simulink library "uav_utilities"  (Simulink 7.1)
values from neighbouring files (symbols this model uses):
  I = find(Ev == Ev(1))    [res_power_junction_m.m]
undefined symbols (not defined in the file or in its folder): euler_0, g, inner_sysd, K_inner, K_outer, Kx_inner, KX_outer, Ky_inner, KY_outer, L, m, omega_0, outer_sysd, pow_gps_pos_sim, pow_gps_vel_sim, pow_imu_pos_sim, pow_imu_rate_sim, pow_sodar_sim, t_comp_inner, t_comp_outer, t_gps, t_imu, t_inner, t_outer, t_sodar, tau, thrust_max, torque_max, Vb_0, XYZ_0
libraries: simulink x33, aero_sim_lib x9, aerolibprivatev1p5 x1
(part 2 of 3)

== system uav_utilities/STARMAC/starmac_dynamics/starmac_motor_dynamics ==
  desired_motor_thrust : Inport  OutDataType=sfix(16)  OutScaling=2^0
  Band-Limited White Noise : simulink/Sources/Band-Limited White Noise  SystemSampleTime=-1  Cov=Ts*motor_variance*ones(4,1)  Ts=Ts  seed=22341+[0 1 2 3]'
  Constant : Constant  Value=motor_lag_enable  OutDataType=sfix(16)  OutScaling=2^0
  Saturation : Saturate  UpperLimit=thrust_max*ones(4,1)  LowerLimit=thrust_min*ones(4,1)
  State-Space : StateSpace  A=-(1/tau_motor)*eye(4)  B=(1/tau_motor)*eye(4)  C=eye(4)  D=zeros(4,4)  X0=T_nom*ones(4,1)
  Sum : Sum  Inputs=|++  OutDataType=sfix(16)  OutScaling=2^0
  Switch : Switch  Criteria=u2 > Threshold  OutDataType=sfix(16)  OutScaling=2^0
  motor_thrust : Outport  OutDataType=sfix(16)  OutScaling=2^0
  wires:
  Constant/1 -> Switch/2
  Switch/1 -> Saturation/1
  State-Space/1 -> Switch/1
  Band-Limited White Noise/1 -> Sum/2
  Saturation/1 -> Sum/1
  Sum/1 -> motor_thrust/1
  desired_motor_thrust/1 -> Switch/3, State-Space/1

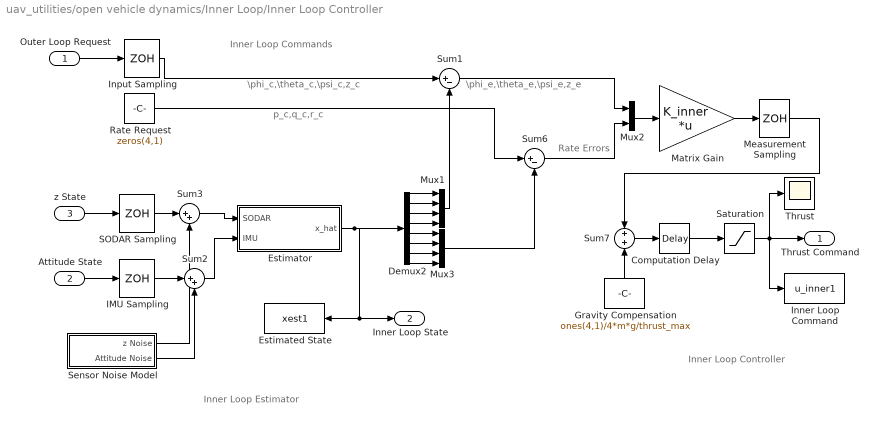
== system uav_utilities/open vehicle dynamics/Inner Loop/Inner Loop Controller ==
  note: \phi_e,\theta_e,\psi_e,z_e
  note: Rate Errors
  note: \phi_c,\theta_c,\psi_c,z_c
  note: Inner Loop Controller
  note: p_c,q_c,r_c
  note: Inner Loop Estimator
  note: Inner Loop Commands
  Outer Loop Request : Inport  OutDataType=sfix(16)  OutScaling=2^0
  Attitude State : Inport  Port=2  OutDataType=sfix(16)  OutScaling=2^0
  z State : Inport  Port=3  OutDataType=sfix(16)  OutScaling=2^0
  Computation Delay : TransportDelay  DelayTime=t_comp_inner  PadeOrder=10
  Demux2 : Demux  Outputs=8
  Estimated State : ToWorkspace  VariableName=xest1  SampleTime=-1  SaveFormat=Array
  Estimator : Subsystem
  Gravity Compensation : Constant  Orientation=up  Value=ones(4,1)/4*m*g/thrust_max  OutDataType=sfix(16)  OutScaling=2^0
  IMU Sampling : ZeroOrderHold  SampleTime=t_imu
  Inner Loop Command : ToWorkspace  VariableName=u_inner1  SampleTime=-1  SaveFormat=Array
  Input Sampling : ZeroOrderHold  SampleTime=t_inner
  Matrix Gain : Gain  Gain=K_inner  Multiplication=Matrix(K*u)  ParameterDataType=sfix(16)  ParameterScaling=2^0  OutDataType=sfix(16)  OutScaling=2^0  SaturateOnIntegerOverflow=on  OutDataTypeStr=Inherit: Same as input  ParamDataTypeStr=Inherit: Same as input
  Measurement Sampling : ZeroOrderHold  SampleTime=t_inner
  Mux1 : Mux
  Mux2 : Mux  Inputs=2
  Mux3 : Mux
  Rate Request : Constant  Value=zeros(4,1)  OutDataType=sfix(16)  OutScaling=2^0
  SODAR Sampling : ZeroOrderHold  SampleTime=t_sodar
  Saturation : Saturate  UpperLimit=1  LowerLimit=0
  "Sensor Noise Model  " : Subsystem
  Sum1 : Sum  Inputs=|+-  OutDataType=sfix(16)  OutScaling=2^0  SaturateOnIntegerOverflow=on
  Sum2 : Sum  Inputs=|++  OutDataType=sfix(16)  OutScaling=2^0  SaturateOnIntegerOverflow=on
  Sum3 : Sum  Inputs=|++  OutDataType=sfix(16)  OutScaling=2^0  SaturateOnIntegerOverflow=on
  Sum6 : Sum  Inputs=|+-  OutDataType=sfix(16)  OutScaling=2^0  SaturateOnIntegerOverflow=on
  Sum7 : Sum  OutDataType=sfix(16)  OutScaling=2^0  SaturateOnIntegerOverflow=on
  Thrust : Scope
      settings: SaveName=ScopeData7
  Thrust Command : Outport  OutDataType=sfix(16)  OutScaling=2^0
  Inner Loop State : Outport  Port=2  OutDataType=sfix(16)  OutScaling=2^0
  wires:
  Attitude State/1 -> IMU Sampling/1
  Sum1/1 -> Mux2/1
  Mux2/1 -> Matrix Gain/1
  Matrix Gain/1 -> Measurement Sampling/1
  z State/1 -> SODAR Sampling/1
  Mux1/1 -> Sum1/2
  Gravity Compensation/1 -> Sum7/2
  Sum7/1 -> Computation Delay/1
  Outer Loop Request/1 -> Input Sampling/1
  Input Sampling/1 -> Sum1/1
  Measurement Sampling/1 -> Sum7/1
  Demux2/3 -> Mux1/3
  Demux2/2 -> Mux1/2
  Demux2/1 -> Mux1/1
  Demux2/4 -> Mux1/4
  Sum6/1 -> Mux2/2
  Rate Request/1 -> Sum6/1
  Mux3/1 -> Sum6/2
  Demux2/5 -> Mux3/1
  Demux2/6 -> Mux3/2
  Demux2/7 -> Mux3/3
  Demux2/8 -> Mux3/4
  Estimator/1(x_hat) -> Demux2/1, Estimated State/1, Inner Loop State/1
  Sum2/1 -> Estimator/2(IMU)
  SODAR Sampling/1 -> Sum3/1
  Sum3/1 -> Estimator/1(SODAR)
  IMU Sampling/1 -> Sum2/1
  Saturation/1 -> Thrust Command/1, Inner Loop Command/1, Thrust/1
  Computation Delay/1 -> Saturation/1
  "Sensor Noise Model  "/1(z Noise) -> Sum3/2
  "Sensor Noise Model  "/2(Attitude Noise) -> Sum2/2

== system uav_utilities/open vehicle dynamics/Inner Loop/Non-Linear Dynamics ==
  Thrust Command 1-4 : Inport  OutDataType=sfix(16)  OutScaling=2^0
  6DOF (Euler Angles)_CMU : aero_sim_lib/6DOF (Euler Angles)_CMU  SystemSampleTime=-1  XYZe_0=XYZ_0  Vb_0=Vb_0  euler_0=euler_0  omega_0=omega_0  M=m  I=I
  Gravity : Constant  Value=[0;0;-m*g]  OutDataType=sfix(16)  OutScaling=2^0
  Motor Model : Subsystem
  Rotational Torques : Subsystem
  Sum : Sum  Inputs=|++  OutDataType=sfix(16)  OutScaling=2^0  SaturateOnIntegerOverflow=on
  Terminator : Terminator
  Terminator1 : Terminator
  Terminator2 : Terminator
  "Body vel " : Outport  OutDataType=sfix(16)  OutScaling=2^0
  Position : Outport  Port=2  OutDataType=sfix(16)  OutScaling=2^0
  Velocity : Outport  Port=3  OutDataType=sfix(16)  OutScaling=2^0
  Angular Rates : Outport  Port=4  OutDataType=sfix(16)  OutScaling=2^0
  Euler Angles : Outport  Port=5  OutDataType=sfix(16)  OutScaling=2^0
  wires:
  Thrust Command 1-4/1 -> Motor Model/1(Thrust Command 1-4), Rotational Torques/1(Thrust Command 1-4)
  Rotational Torques/1(Moments) -> 6DOF (Euler Angles)_CMU/2
  6DOF (Euler Angles)_CMU/1 -> Velocity/1
  6DOF (Euler Angles)_CMU/2 -> Position/1
  6DOF (Euler Angles)_CMU/5 -> "Body vel "/1
  6DOF (Euler Angles)_CMU/3 -> Motor Model/2(Euler (rad)), Euler Angles/1
  6DOF (Euler Angles)_CMU/6 -> Angular Rates/1
  6DOF (Euler Angles)_CMU/4 -> Terminator1/1
  6DOF (Euler Angles)_CMU/7 -> Terminator/1
  Motor Model/1("Force_b ") -> Sum/1
  Gravity/1 -> Sum/2
  Sum/1 -> 6DOF (Euler Angles)_CMU/1
  6DOF (Euler Angles)_CMU/8 -> Terminator2/1

== system uav_utilities/open vehicle dynamics/Inner Loop/Saturation ==
  note: No longer saturating
      | the z cordinate??!!!XXX
      | was set from 0 to 3
      | Nicholas Kottenstette
  Actual : Inport  OutDataType=sfix(16)  OutScaling=2^0
  Demux : Demux  Outputs=3
  Mux : Mux  Inputs=3
  Sensed : Outport  OutDataType=sfix(16)  OutScaling=2^0
  wires:
  Actual/1 -> Demux/1
  Mux/1 -> Sensed/1
  Demux/2 -> Mux/2
  Demux/1 -> Mux/1
  Demux/3 -> Mux/3

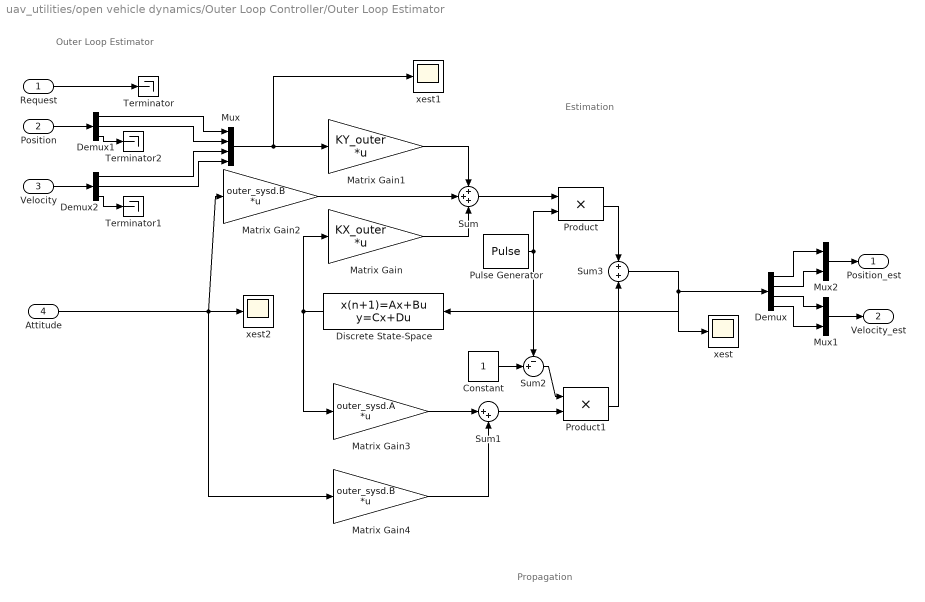
== system uav_utilities/open vehicle dynamics/Outer Loop Controller/Outer Loop Estimator ==
  note: Outer Loop Estimator
  note: Estimation
  note: Propagation
  Request : Inport  OutDataType=sfix(16)  OutScaling=2^0
  Position : Inport  Port=2  OutDataType=sfix(16)  OutScaling=2^0
  Velocity : Inport  Port=3  OutDataType=sfix(16)  OutScaling=2^0
  Attitude : Inport  Port=4  OutDataType=sfix(16)  OutScaling=2^0
  Constant : Constant  OutDataType=sfix(16)  OutScaling=2^0
  Demux : Demux
  Demux1 : Demux  Outputs=3
  Demux2 : Demux  Outputs=3
  Discrete State-Space : DiscreteStateSpace  Orientation=left  A=zeros(4)  B=eye(4)  C=eye(4)  D=zeros(4)  X0=zeros(4,1)  SampleTime=t_outer
  Matrix Gain : Gain  Gain=KX_outer  Multiplication=Matrix(K*u)  ParameterDataType=sfix(16)  ParameterScaling=2^0  OutDataType=sfix(16)  OutScaling=2^0  SaturateOnIntegerOverflow=on  OutDataTypeStr=Inherit: Same as input  ParamDataTypeStr=Inherit: Same as input
  Matrix Gain1 : Gain  Gain=KY_outer  Multiplication=Matrix(K*u)  ParameterDataType=sfix(16)  ParameterScaling=2^0  OutDataType=sfix(16)  OutScaling=2^0  SaturateOnIntegerOverflow=on  OutDataTypeStr=Inherit: Same as input  ParamDataTypeStr=Inherit: Same as input
  Matrix Gain2 : Gain  Gain=outer_sysd.B  Multiplication=Matrix(K*u)  ParameterDataType=sfix(16)  ParameterScaling=2^0  OutDataType=sfix(16)  OutScaling=2^0  SaturateOnIntegerOverflow=on  OutDataTypeStr=Inherit: Same as input  ParamDataTypeStr=Inherit: Same as input
  Matrix Gain3 : Gain  Gain=outer_sysd.A  Multiplication=Matrix(K*u)  ParameterDataType=sfix(16)  ParameterScaling=2^0  OutDataType=sfix(16)  OutScaling=2^0  SaturateOnIntegerOverflow=on  OutDataTypeStr=Inherit: Same as input  ParamDataTypeStr=Inherit: Same as input
  Matrix Gain4 : Gain  Gain=outer_sysd.B  Multiplication=Matrix(K*u)  ParameterDataType=sfix(16)  ParameterScaling=2^0  OutDataType=sfix(16)  OutScaling=2^0  SaturateOnIntegerOverflow=on  OutDataTypeStr=Inherit: Same as input  ParamDataTypeStr=Inherit: Same as input
  Mux : Mux
  Mux1 : Mux  Inputs=2
  Mux2 : Mux  Inputs=2
  Product : Product  OutDataType=sfix(16)  OutScaling=2^0  SaturateOnIntegerOverflow=on  OutDataTypeStr=Inherit: Same as first input
  Product1 : Product  OutDataType=sfix(16)  OutScaling=2^0  SaturateOnIntegerOverflow=on  OutDataTypeStr=Inherit: Same as first input
  Pulse Generator : DiscretePulseGenerator  PulseType=Time based  Period=t_gps  PulseWidth=100*t_outer/t_gps
  Sum : Sum  Inputs=+++  OutDataType=sfix(16)  OutScaling=2^0  SaturateOnIntegerOverflow=on
  Sum1 : Sum  Inputs=|++  OutDataType=sfix(16)  OutScaling=2^0  SaturateOnIntegerOverflow=on
  Sum2 : Sum  Inputs=-+|  OutDataType=sfix(16)  OutScaling=2^0  SaturateOnIntegerOverflow=on
  Sum3 : Sum  OutDataType=sfix(16)  OutScaling=2^0  SaturateOnIntegerOverflow=on
  Terminator : Terminator
  Terminator1 : Terminator
  Terminator2 : Terminator
  xest : Scope
      settings: Decimation=10
  xest1 : Scope
      settings: SaveName=ScopeData9  Decimation=10
  xest2 : Scope
      settings: SaveName=ScopeData10
  Position_est : Outport  OutDataType=sfix(16)  OutScaling=2^0
  Velocity_est : Outport  Port=2  OutDataType=sfix(16)  OutScaling=2^0
  wires:
  Request/1 -> Terminator/1
  Matrix Gain1/1 -> Sum/1
  Sum/1 -> Product/1
  Matrix Gain/1 -> Sum/3
  Matrix Gain2/1 -> Sum/2
  Discrete State-Space/1 -> Matrix Gain/1, Matrix Gain3/1
  Mux/1 -> Matrix Gain1/1, xest1/1
  Mux1/1 -> Velocity_est/1
  Mux2/1 -> Position_est/1
  Demux/1 -> Mux2/1
  Demux/2 -> Mux2/2
  Demux/3 -> Mux1/1
  Demux/4 -> Mux1/2
  Position/1 -> Demux1/1
  Velocity/1 -> Demux2/1
  Demux2/3 -> Terminator1/1
  Demux1/3 -> Terminator2/1
  Demux2/1 -> Mux/3
  Demux2/2 -> Mux/4
  Demux1/2 -> Mux/2
  Demux1/1 -> Mux/1
  Attitude/1 -> Matrix Gain2/1, xest2/1, Matrix Gain4/1
  Matrix Gain4/1 -> Sum1/2
  Matrix Gain3/1 -> Sum1/1
  Pulse Generator/1 -> Product/2, Sum2/1
  Product/1 -> Sum3/1
  Constant/1 -> Sum2/2
  Sum2/1 -> Product1/1
  Sum1/1 -> Product1/2
  Product1/1 -> Sum3/2
  Sum3/1 -> Demux/1, Discrete State-Space/1, xest/1

== system uav_utilities/open vehicle dynamics/Outer Loop Controller/Sensor Noise Model  ==
  Mux1 : Mux  Inputs=3
  Mux3 : Mux  Inputs=3
  Vx White Noise : simulink/Sources/Band-Limited White Noise  SystemSampleTime=-1  Cov=[pow_gps_vel_sim]  Ts=t_gps  seed=[2]
  Vy White Noise : simulink/Sources/Band-Limited White Noise  SystemSampleTime=-1  Cov=[pow_gps_vel_sim]  Ts=t_gps  seed=[500]
  Vz White Noise : simulink/Sources/Band-Limited White Noise  SystemSampleTime=-1  Cov=[pow_gps_vel_sim]  Ts=t_gps  seed=[1000]
  x White Noise : simulink/Sources/Band-Limited White Noise  SystemSampleTime=-1  Cov=[pow_gps_pos_sim]  Ts=t_gps  seed=[13341]
  y White Noise : simulink/Sources/Band-Limited White Noise  SystemSampleTime=-1  Cov=[pow_gps_pos_sim]  Ts=t_gps  seed=[23121]
  z White Noise1 : simulink/Sources/Band-Limited White Noise  SystemSampleTime=-1  Cov=[pow_gps_pos_sim]  Ts=t_gps  seed=[53341]
  Position Noise : Outport  OutDataType=sfix(16)  OutScaling=2^0
  Velocity Noise : Outport  Port=2  OutDataType=sfix(16)  OutScaling=2^0
  wires:
  Mux3/1 -> Position Noise/1
  z White Noise1/1 -> Mux3/3
  y White Noise/1 -> Mux3/2
  x White Noise/1 -> Mux3/1
  Mux1/1 -> Velocity Noise/1
  Vz White Noise/1 -> Mux1/3
  Vy White Noise/1 -> Mux1/2
  Vx White Noise/1 -> Mux1/1

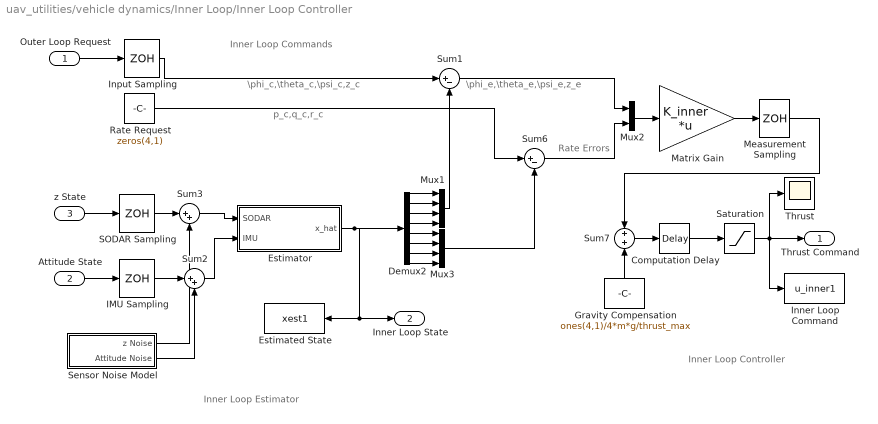
== system uav_utilities/vehicle dynamics/Inner Loop/Inner Loop Controller ==
  note: Inner Loop Commands
  note: Inner Loop Estimator
  note: p_c,q_c,r_c
  note: Inner Loop Controller
  note: \phi_c,\theta_c,\psi_c,z_c
  note: Rate Errors
  note: \phi_e,\theta_e,\psi_e,z_e
  Outer Loop Request : Inport
  Attitude State : Inport  Port=2
  z State : Inport  Port=3
  Computation Delay : TransportDelay  DelayTime=t_comp_inner  PadeOrder=10
  Demux2 : Demux  Outputs=8
  Estimated State : ToWorkspace  VariableName=xest1  SampleTime=-1  SaveFormat=Array
  Estimator : Subsystem
  Gravity Compensation : Constant  Orientation=up  Value=ones(4,1)/4*m*g/thrust_max
  IMU Sampling : ZeroOrderHold  SampleTime=t_imu
  Inner Loop Command : ToWorkspace  VariableName=u_inner1  SampleTime=-1  SaveFormat=Array
  Input Sampling : ZeroOrderHold  SampleTime=t_inner
  Matrix Gain : Gain  Gain=K_inner  Multiplication=Matrix(K*u)  SaturateOnIntegerOverflow=on  OutDataTypeStr=Inherit: Same as input  ParamDataTypeStr=Inherit: Same as input
  Measurement Sampling : ZeroOrderHold  SampleTime=t_inner
  Mux1 : Mux
  Mux2 : Mux  Inputs=2
  Mux3 : Mux
  Rate Request : Constant  Value=zeros(4,1)
  SODAR Sampling : ZeroOrderHold  SampleTime=t_sodar
  Saturation : Saturate  UpperLimit=1  LowerLimit=0
  "Sensor Noise Model  " : Subsystem
  Sum1 : Sum  Inputs=|+-  SaturateOnIntegerOverflow=on
  Sum2 : Sum  Inputs=|++  SaturateOnIntegerOverflow=on
  Sum3 : Sum  Inputs=|++  SaturateOnIntegerOverflow=on
  Sum6 : Sum  Inputs=|+-  SaturateOnIntegerOverflow=on
  Sum7 : Sum  SaturateOnIntegerOverflow=on
  Thrust : Scope
      settings: SaveName=ScopeData7
  Thrust Command : Outport
  Inner Loop State : Outport  Port=2
  wires:
  "Sensor Noise Model  "/2(Attitude Noise) -> Sum2/2
  "Sensor Noise Model  "/1(z Noise) -> Sum3/2
  Computation Delay/1 -> Saturation/1
  Saturation/1 -> Thrust/1, Inner Loop Command/1, Thrust Command/1
  IMU Sampling/1 -> Sum2/1
  Sum3/1 -> Estimator/1(SODAR)
  SODAR Sampling/1 -> Sum3/1
  Sum2/1 -> Estimator/2(IMU)
  Estimator/1(x_hat) -> Inner Loop State/1, Estimated State/1, Demux2/1
  Demux2/8 -> Mux3/4
  Demux2/7 -> Mux3/3
  Demux2/6 -> Mux3/2
  Demux2/5 -> Mux3/1
  Mux3/1 -> Sum6/2
  Rate Request/1 -> Sum6/1
  Sum6/1 -> Mux2/2
  Demux2/4 -> Mux1/4
  Demux2/1 -> Mux1/1
  Demux2/2 -> Mux1/2
  Demux2/3 -> Mux1/3
  Measurement Sampling/1 -> Sum7/1
  Input Sampling/1 -> Sum1/1
  Outer Loop Request/1 -> Input Sampling/1
  Sum7/1 -> Computation Delay/1
  Gravity Compensation/1 -> Sum7/2
  Mux1/1 -> Sum1/2
  z State/1 -> SODAR Sampling/1
  Matrix Gain/1 -> Measurement Sampling/1
  Mux2/1 -> Matrix Gain/1
  Sum1/1 -> Mux2/1
  Attitude State/1 -> IMU Sampling/1

== system uav_utilities/vehicle dynamics/Inner Loop/Non-Linear Dynamics ==
  Thrust Command 1-4 : Inport
  6DoF (Quaternion) : aerolibprivatev1p5/6DoF (Quaternion)  SystemSampleTime=-1  xme_0=XYZ_0'  Vm_0=Vb_0'  eul_0=euler_0'  pm_0=omega_0'  Mass=m  Inertia=I  k_quat=1
  Gravity : Constant  Value=[0;0;-m*g]
  Motor Model : Subsystem
  Rotational Torques : Subsystem
  Sum : Sum  Inputs=|++  SaturateOnIntegerOverflow=on
  Terminator : Terminator
  Terminator1 : Terminator
  "Body vel " : Outport
  Position : Outport  Port=2
  Velocity : Outport  Port=3
  Angular Rates : Outport  Port=4
  Euler Angles : Outport  Port=5
  wires:
  Sum/1 -> 6DoF (Quaternion)/1
  Gravity/1 -> Sum/2
  Motor Model/1("Force_b ") -> Sum/1
  6DoF (Quaternion)/7 -> Terminator/1
  6DoF (Quaternion)/4 -> Terminator1/1
  6DoF (Quaternion)/6 -> Angular Rates/1
  6DoF (Quaternion)/3 -> Euler Angles/1, Motor Model/2(Euler (rad))
  6DoF (Quaternion)/5 -> "Body vel "/1
  6DoF (Quaternion)/2 -> Position/1
  6DoF (Quaternion)/1 -> Velocity/1
  Rotational Torques/1(Moments) -> 6DoF (Quaternion)/2
  Thrust Command 1-4/1 -> Rotational Torques/1(Thrust Command 1-4), Motor Model/1(Thrust Command 1-4)

== system uav_utilities/vehicle dynamics/Inner Loop/Saturation ==
  note: No longer saturating
      | the z cordinate??!!!XXX
      | was set from 0 to 3
      | Nicholas Kottenstette
  Actual : Inport
  Demux : Demux  Outputs=3
  Mux : Mux  Inputs=3
  Sensed : Outport
  wires:
  Demux/3 -> Mux/3
  Demux/1 -> Mux/1
  Demux/2 -> Mux/2
  Mux/1 -> Sensed/1
  Actual/1 -> Demux/1

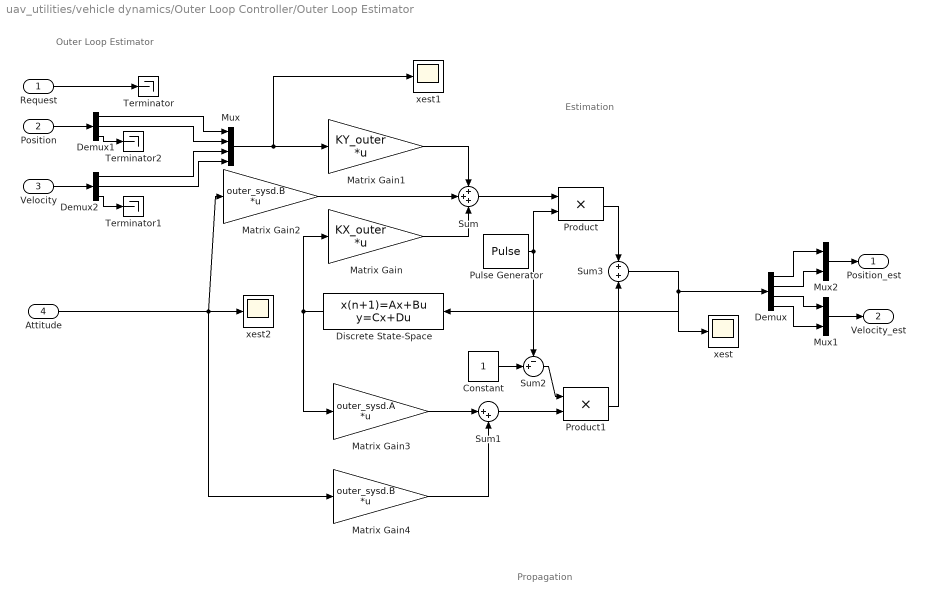
== system uav_utilities/vehicle dynamics/Outer Loop Controller/Outer Loop Estimator ==
  note: Propagation
  note: Estimation
  note: Outer Loop Estimator
  Request : Inport
  Position : Inport  Port=2
  Velocity : Inport  Port=3
  Attitude : Inport  Port=4
  Constant : Constant
  Demux : Demux
  Demux1 : Demux  Outputs=3
  Demux2 : Demux  Outputs=3
  Discrete State-Space : DiscreteStateSpace  Orientation=left  A=zeros(4)  B=eye(4)  C=eye(4)  D=zeros(4)  X0=zeros(4,1)  SampleTime=t_outer
  Matrix Gain : Gain  Gain=KX_outer  Multiplication=Matrix(K*u)  SaturateOnIntegerOverflow=on  OutDataTypeStr=Inherit: Same as input  ParamDataTypeStr=Inherit: Same as input
  Matrix Gain1 : Gain  Gain=KY_outer  Multiplication=Matrix(K*u)  SaturateOnIntegerOverflow=on  OutDataTypeStr=Inherit: Same as input  ParamDataTypeStr=Inherit: Same as input
  Matrix Gain2 : Gain  Gain=outer_sysd.B  Multiplication=Matrix(K*u)  SaturateOnIntegerOverflow=on  OutDataTypeStr=Inherit: Same as input  ParamDataTypeStr=Inherit: Same as input
  Matrix Gain3 : Gain  Gain=outer_sysd.A  Multiplication=Matrix(K*u)  SaturateOnIntegerOverflow=on  OutDataTypeStr=Inherit: Same as input  ParamDataTypeStr=Inherit: Same as input
  Matrix Gain4 : Gain  Gain=outer_sysd.B  Multiplication=Matrix(K*u)  SaturateOnIntegerOverflow=on  OutDataTypeStr=Inherit: Same as input  ParamDataTypeStr=Inherit: Same as input
  Mux : Mux
  Mux1 : Mux  Inputs=2
  Mux2 : Mux  Inputs=2
  Product : Product  SaturateOnIntegerOverflow=on  OutDataTypeStr=Inherit: Same as first input
  Product1 : Product  SaturateOnIntegerOverflow=on  OutDataTypeStr=Inherit: Same as first input
  Pulse Generator : DiscretePulseGenerator  PulseType=Time based  Period=t_gps  PulseWidth=100*t_outer/t_gps
  Sum : Sum  Inputs=+++  SaturateOnIntegerOverflow=on
  Sum1 : Sum  Inputs=|++  SaturateOnIntegerOverflow=on
  Sum2 : Sum  Inputs=-+|  SaturateOnIntegerOverflow=on
  Sum3 : Sum  SaturateOnIntegerOverflow=on
  Terminator : Terminator
  Terminator1 : Terminator
  Terminator2 : Terminator
  xest : Scope
      settings: Decimation=10
  xest1 : Scope
      settings: SaveName=ScopeData9  Decimation=10
  xest2 : Scope
      settings: SaveName=ScopeData10
  Position_est : Outport
  Velocity_est : Outport  Port=2
  wires:
  Sum3/1 -> xest/1, Discrete State-Space/1, Demux/1
  Product1/1 -> Sum3/2
  Sum1/1 -> Product1/2
  Sum2/1 -> Product1/1
  Constant/1 -> Sum2/2
  Product/1 -> Sum3/1
  Pulse Generator/1 -> Sum2/1, Product/2
  Matrix Gain3/1 -> Sum1/1
  Matrix Gain4/1 -> Sum1/2
  Attitude/1 -> Matrix Gain4/1, xest2/1, Matrix Gain2/1
  Demux1/1 -> Mux/1
  Demux1/2 -> Mux/2
  Demux2/2 -> Mux/4
  Demux2/1 -> Mux/3
  Demux1/3 -> Terminator2/1
  Demux2/3 -> Terminator1/1
  Velocity/1 -> Demux2/1
  Position/1 -> Demux1/1
  Demux/4 -> Mux1/2
  Demux/3 -> Mux1/1
  Demux/2 -> Mux2/2
  Demux/1 -> Mux2/1
  Mux2/1 -> Position_est/1
  Mux1/1 -> Velocity_est/1
  Mux/1 -> xest1/1, Matrix Gain1/1
  Discrete State-Space/1 -> Matrix Gain3/1, Matrix Gain/1
  Matrix Gain2/1 -> Sum/2
  Matrix Gain/1 -> Sum/3
  Sum/1 -> Product/1
  Matrix Gain1/1 -> Sum/1
  Request/1 -> Terminator/1

== system uav_utilities/vehicle dynamics/Outer Loop Controller/Sensor Noise Model  ==
  Mux1 : Mux  Inputs=3
  Mux3 : Mux  Inputs=3
  Vx White Noise : simulink/Sources/Band-Limited White Noise  SystemSampleTime=-1  Cov=[pow_gps_vel_sim]  Ts=t_gps  seed=[2]
  Vy White Noise : simulink/Sources/Band-Limited White Noise  SystemSampleTime=-1  Cov=[pow_gps_vel_sim]  Ts=t_gps  seed=[500]
  Vz White Noise : simulink/Sources/Band-Limited White Noise  SystemSampleTime=-1  Cov=[pow_gps_vel_sim]  Ts=t_gps  seed=[1000]
  x White Noise : simulink/Sources/Band-Limited White Noise  SystemSampleTime=-1  Cov=[pow_gps_pos_sim]  Ts=t_gps  seed=[13341]
  y White Noise : simulink/Sources/Band-Limited White Noise  SystemSampleTime=-1  Cov=[pow_gps_pos_sim]  Ts=t_gps  seed=[23121]
  z White Noise1 : simulink/Sources/Band-Limited White Noise  SystemSampleTime=-1  Cov=[pow_gps_pos_sim]  Ts=t_gps  seed=[53341]
  Position Noise : Outport
  Velocity Noise : Outport  Port=2
  wires:
  Vx White Noise/1 -> Mux1/1
  Vy White Noise/1 -> Mux1/2
  Vz White Noise/1 -> Mux1/3
  Mux1/1 -> Velocity Noise/1
  x White Noise/1 -> Mux3/1
  y White Noise/1 -> Mux3/2
  z White Noise1/1 -> Mux3/3
  Mux3/1 -> Position Noise/1

== system uav_utilities/STARMAC/gum_stix/body_to_inertial/inertial_vel_and pos_est ==
  Ab : Inport
  DT_integrator : Subsystem
  DT_integrator1 : Subsystem
  Vb : Outport
  Xb : Outport  Port=2
  wires:
  DT_integrator/1(Vb) -> DT_integrator1/1(Vb), Vb/1
  Ab/1 -> DT_integrator/1(Ab)
  DT_integrator1/1(Xb) -> Xb/1

== system uav_utilities/STARMAC/gum_stix/inertial_pos_controller/input_filter ==
  yaw_set : Inport  OutDataType=sfix(16)  OutScaling=2^0
  Discrete Transfer Fcn : DiscreteTransferFcn  Numerator=Hz.num{1}  Denominator=Hz.den{1}  SampleTime=-1
  yaw_r : Outport  OutDataType=sfix(16)  OutScaling=2^0
  wires:
  Discrete Transfer Fcn/1 -> yaw_r/1
  yaw_set/1 -> Discrete Transfer Fcn/1

== system uav_utilities/STARMAC/gum_stix/inertial_pos_controller/vel_est ==
  Xe_set : Inport
  Demux : Demux  Outputs=3
  Discrete Transfer Fcn : DiscreteTransferFcn  Numerator=Hz.num{1}  Denominator=Hz.den{1}  SampleTime=-1
  Discrete Transfer Fcn1 : DiscreteTransferFcn  Numerator=Hz.num{1}  Denominator=Hz.den{1}  SampleTime=-1
  Discrete Transfer Fcn2 : DiscreteTransferFcn  Numerator=Hz.num{1}  Denominator=Hz.den{1}  SampleTime=-1
  Mux : Mux  Inputs=3
  Ve_set : Outport
  wires:
  Discrete Transfer Fcn2/1 -> Mux/3
  Discrete Transfer Fcn1/1 -> Mux/2
  Discrete Transfer Fcn/1 -> Mux/1
  Mux/1 -> Ve_set/1
  Demux/3 -> Discrete Transfer Fcn2/1
  Demux/2 -> Discrete Transfer Fcn1/1
  Demux/1 -> Discrete Transfer Fcn/1
  Xe_set/1 -> Demux/1  "x"

== system uav_utilities/STARMAC/gum_stix/sensor_fusion/delays ==
  dV : Inport  Orientation=left
  dX : Inport  Orientation=left  Port=2
  Ve_sh : Inport  Orientation=left  Port=3
  Xe_sh : Inport  Orientation=left  Port=4
  u_delay{,1..3} (4 alike) : UnitDelay  Orientation=left  SampleTime=-1
  dV_1 : Outport  Orientation=left
  dX_1 : Outport  Orientation=left  Port=2
  Ve_sh_1 : Outport  Orientation=left  Port=3
  Xe_sh_1 : Outport  Orientation=left  Port=4
  wires:
  u_delay3/1 -> Xe_sh_1/1
  Xe_sh/1 -> u_delay3/1
  u_delay2/1 -> Ve_sh_1/1
  Ve_sh/1 -> u_delay2/1
  u_delay1/1 -> dX_1/1
  dX/1 -> u_delay1/1
  u_delay/1 -> dV_1/1
  dV/1 -> u_delay/1

== system uav_utilities/STARMAC/gum_stix/sensor_fusion/if_end ==
  Xe_s : Inport
  Xe_f : Inport  Port=2
  dX_1p : Inport  Port=3
  Xe_sh_1p : Inport  Port=4
  If : If  NumInputs=2  IfExpression=(u1(1) ~= u2(1)) | (u1(2) ~= u2(2)) | (u1(3) ~= u2(3))
  If Action Subsystem : Subsystem  TreatAsAtomicUnit=on
  If Action Subsystem1 : Subsystem  TreatAsAtomicUnit=on
  Sum : Sum  Inputs=|++  OutDataTypeMode=single  OutDataType=sfix(16)  OutScaling=2^0  OutDataTypeStr=single
  Sum1 : Sum  Inputs=|++  OutDataTypeMode=single  OutDataType=sfix(16)  OutScaling=2^0  OutDataTypeStr=single
  Xe_sh_1 : Outport
  dX_1 : Outport  Port=2
  wires:
  dX_1p/1 -> If Action Subsystem1/2(dX_1p)
  Sum1/1 -> dX_1/1
  Xe_f/1 -> If Action Subsystem/2(Xe_f)
  Sum/1 -> Xe_sh_1/1
  If Action Subsystem1/2(dX_1) -> Sum1/2
  If Action Subsystem1/1(Xe_sh_1) -> Sum/2
  If Action Subsystem/2(dX_1) -> Sum1/1
  If Action Subsystem/1(Xe_sh_1) -> Sum/1
  Xe_sh_1p/1 -> If Action Subsystem1/1(Xe_sh_1p), If/2
  Xe_s/1 -> If/1, If Action Subsystem/1(Xe_s)
  If/2 -> If Action Subsystem1/Action
  If/1 -> If Action Subsystem/Action

== system uav_utilities/STARMAC/gum_stix/sensor_fusion/if_end1 ==
  Ve_s : Inport
  Ve_f : Inport  Port=2
  dV_1p : Inport  Port=3
  Ve_sh_1p : Inport  Port=4
  If : If  NumInputs=2  IfExpression=(u1(1) ~= u2(1)) | (u1(2) ~= u2(2)) | (u1(3) ~= u2(3))
  If Action Subsystem : Subsystem  TreatAsAtomicUnit=on
  If Action Subsystem1 : Subsystem  TreatAsAtomicUnit=on
  Sum : Sum  Inputs=|++  OutDataTypeMode=single  OutDataType=sfix(16)  OutScaling=2^0  OutDataTypeStr=single
  Sum1 : Sum  Inputs=|++  OutDataTypeMode=single  OutDataType=sfix(16)  OutScaling=2^0  OutDataTypeStr=single
  Ve_sh_1 : Outport
  dV_1 : Outport  Port=2
  wires:
  If/1 -> If Action Subsystem/Action
  If/2 -> If Action Subsystem1/Action
  Ve_s/1 -> If Action Subsystem/1(Ve_s), If/1
  Ve_sh_1p/1 -> If/2, If Action Subsystem1/1(Ve_sh_1p)
  If Action Subsystem/1(Ve_sh_1) -> Sum/1
  If Action Subsystem/2(dV_1) -> Sum1/1
  If Action Subsystem1/1(Ve_sh_1) -> Sum/2
  If Action Subsystem1/2(dV_1) -> Sum1/2
  Sum/1 -> Ve_sh_1/1
  Ve_f/1 -> If Action Subsystem/2(Ve_f)
  Sum1/1 -> dV_1/1
  dV_1p/1 -> If Action Subsystem1/2(dV_1p)

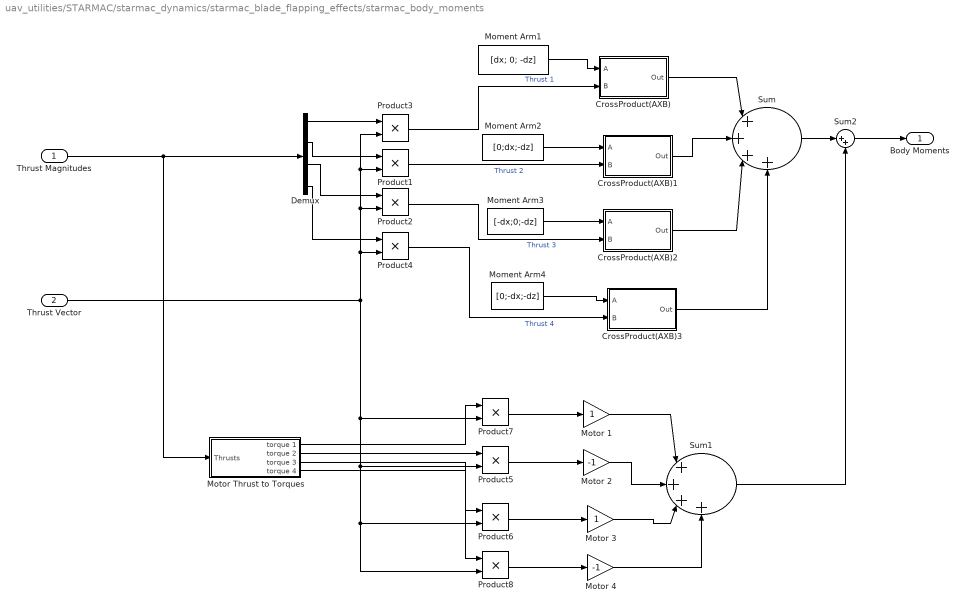
== system uav_utilities/STARMAC/starmac_dynamics/starmac_blade_flapping_effects/starmac_body_moments ==
  Thrust Magnitudes : Inport  OutDataType=sfix(16)  OutScaling=2^0
  Thrust Vector : Inport  Port=2  OutDataType=sfix(16)  OutScaling=2^0
  CrossProduct(AXB) : Subsystem
  CrossProduct(AXB)1 : Subsystem
  CrossProduct(AXB)2 : Subsystem
  CrossProduct(AXB)3 : Subsystem
  Demux : Demux
  Moment Arm1 : Constant  Value=[dx; 0; -dz]  OutDataType=sfix(16)  OutScaling=2^0
  Moment Arm2 : Constant  Value=[0;dx;-dz]  OutDataType=sfix(16)  OutScaling=2^0
  Moment Arm3 : Constant  Value=[-dx;0;-dz]  OutDataType=sfix(16)  OutScaling=2^0
  Moment Arm4 : Constant  Value=[0;-dx;-dz]  OutDataType=sfix(16)  OutScaling=2^0
  Motor 1 : Gain  ParameterDataType=sfix(16)  ParameterScaling=2^0  OutDataType=sfix(16)  OutScaling=2^0
  Motor 2 : Gain  Gain=-1  ParameterDataType=sfix(16)  ParameterScaling=2^0  OutDataType=sfix(16)  OutScaling=2^0
  Motor 3 : Gain  ParameterDataType=sfix(16)  ParameterScaling=2^0  OutDataType=sfix(16)  OutScaling=2^0
  Motor 4 : Gain  Gain=-1  ParameterDataType=sfix(16)  ParameterScaling=2^0  OutDataType=sfix(16)  OutScaling=2^0
  Motor Thrust to Torques : Subsystem
  Product{1..8} (8 alike) : Product  OutDataType=sfix(16)  OutScaling=2^0  RndMeth=Zero
  Sum : Sum  Inputs=|++++  OutDataType=sfix(16)  OutScaling=2^0
  Sum1 : Sum  Inputs=|++++  OutDataType=sfix(16)  OutScaling=2^0
  Sum2 : Sum  Inputs=|++  OutDataType=sfix(16)  OutScaling=2^0
  Body Moments : Outport  OutDataType=sfix(16)  OutScaling=2^0
  wires:
  Thrust Magnitudes/1 -> Demux/1, Motor Thrust to Torques/1(Thrusts)
  Demux/1 -> Product3/1
  Demux/2 -> Product1/1
  Demux/3 -> Product2/1
  Demux/4 -> Product4/1
  Thrust Vector/1 -> Product3/2, Product1/2, Product2/2, Product4/2, Product7/2, Product5/2, Product6/2, Product8/2
  Moment Arm1/1 -> CrossProduct(AXB)/1(A)
  Product3/1 -> CrossProduct(AXB)/2(B)  "Thrust 1"
  Moment Arm2/1 -> CrossProduct(AXB)1/1(A)
  Product1/1 -> CrossProduct(AXB)1/2(B)  "Thrust 2"
  Moment Arm3/1 -> CrossProduct(AXB)2/1(A)
  Product2/1 -> CrossProduct(AXB)2/2(B)  "Thrust 3"
  Moment Arm4/1 -> CrossProduct(AXB)3/1(A)
  Product4/1 -> CrossProduct(AXB)3/2(B)  "Thrust 4"
  CrossProduct(AXB)/1(Out) -> Sum/1
  CrossProduct(AXB)2/1(Out) -> Sum/3
  CrossProduct(AXB)3/1(Out) -> Sum/4
  Motor 1/1 -> Sum1/1
  Motor 2/1 -> Sum1/2
  Motor 3/1 -> Sum1/3
  Motor 4/1 -> Sum1/4
  Sum/1 -> Sum2/1
  Sum1/1 -> Sum2/2
  Sum2/1 -> Body Moments/1
  Product7/1 -> Motor 1/1
  Product5/1 -> Motor 2/1
  Product6/1 -> Motor 3/1
  Product8/1 -> Motor 4/1
  Motor Thrust to Torques/1(torque 1) -> Product7/1
  Motor Thrust to Torques/2(torque 2) -> Product5/1
  Motor Thrust to Torques/3(torque 3) -> Product6/1
  Motor Thrust to Torques/4(torque 4) -> Product8/1
  CrossProduct(AXB)1/1(Out) -> Sum/2

== system uav_utilities/STARMAC/starmac_dynamics/starmac_blade_flapping_effects/starmac_flapping_dynamics ==
  Vb2_hat : Inport  OutDataType=sfix(16)  OutScaling=2^0
  "Body Z " : Constant  Value=[0; 0; -1];  OutDataType=sfix(16)  OutScaling=2^0
  Constant : Constant  OutDataType=sfix(16)  OutScaling=2^0
  Divide : Product  Inputs=*/  OutDataType=sfix(16)  OutScaling=2^-10
  Dot Product : simulink/Math Operations/Dot Product  InputSameDT=on  OutDataType=sfix(16)  OutScaling=2^-10  DoSatur=off
  Flap Angle Gain : Gain  Gain=K_a1s  ParameterDataType=sfix(16)  ParameterScaling=2^0  OutDataType=sfix(16)  OutScaling=2^0
  Gain : Gain  Gain=-1  ParameterDataType=sfix(16)  ParameterScaling=2^0  OutDataType=sfix(16)  OutScaling=2^0
  Gain1 : Gain  Gain=K_beta  ParameterDataType=sfix(16)  ParameterScaling=2^0  OutDataType=sfix(16)  OutScaling=2^0
  Gain2 : Gain  Gain=4  ParameterDataType=sfix(16)  ParameterScaling=2^0  OutDataType=sfix(16)  OutScaling=2^0
  Math Function : Math  Operator=sqrt  OutDataType=sfix(16)  OutScaling=2^0  SaturateOnIntegerOverflow=on
  Product{1..4} (4 alike) : Product  OutDataType=sfix(16)  OutScaling=2^0  RndMeth=Zero
  Sum : Sum  Inputs=|++  OutDataType=sfix(16)  OutScaling=2^0
  Sum1 : Sum  Inputs=|++  OutDataType=sfix(16)  OutScaling=2^0
  Trigonometric Function : Trigonometry
  Trigonometric Function1 : Trigonometry  Operator=cos
  minor_offset : Constant  Value=.001  OutDataType=sfix(16)  OutScaling=2^0
  rotate 90 degrees : Gain  Gain=[0 -1 0;1 0 0;0 0 1]  Multiplication=Matrix(K*u)  ParameterDataType=sfix(16)  ParameterScaling=2^0  OutDataType=sfix(16)  OutScaling=2^0
  thrust_vector : Outport  OutDataType=sfix(16)  OutScaling=2^0
  rotor_blade_moments : Outport  Port=2  OutDataType=sfix(16)  OutScaling=2^0
  wires:
  Constant/1 -> Product4/1
  Flap Angle Gain/1 -> Product4/2
  Gain1/1 -> Product2/1
  rotate 90 degrees/1 -> Product2/2
  Product2/1 -> Gain2/1
  Gain2/1 -> rotor_blade_moments/1
  Sum/1 -> thrust_vector/1
  "Body Z "/1 -> Product1/1
  Product1/1 -> Sum/1
  Gain/1 -> Product3/2
  Product3/1 -> Sum/2
  Trigonometric Function/1 -> Product3/1
  Trigonometric Function1/1 -> Product1/2
  Math Function/1 -> Flap Angle Gain/1, Sum1/1  "v"
  Dot Product/1 -> Math Function/1
  Vb2_hat/1 -> Dot Product/2, Dot Product/1, Divide/1
  Product4/1 -> Gain1/1, Trigonometric Function/1, Trigonometric Function1/1  "flap angle"
  Divide/1 -> Gain/1, rotate 90 degrees/1  "unit vector"
  Sum1/1 -> Divide/2
  minor_offset/1 -> Sum1/2

== system uav_utilities/STARMAC/starmac_dynamics/starmac_blade_flapping_effects/starmac_vertical_effect_dynamics ==
  motor_thrusts : Inport  OutDataType=sfix(16)  OutScaling=2^0
  v_body_relative : Inport  Port=2  OutDataType=sfix(16)  OutScaling=2^0
  Demux : Demux
  Mux : Mux
  starmac_motor_vertical_effect_dynamics{,1..3} (4 alike) : aero_sim_lib/starmac_motor_vertical_effect_dynamics  SystemSampleTime=-1  tau_motor=tau_motor  R=R  Alpha=Alpha  Vinf=Vinf  Vh=Vh  ToverTh=ToverTh
  thrust_multiplier : Outport  OutDataType=sfix(16)  OutScaling=2^0
  wires:
  v_body_relative/1 -> starmac_motor_vertical_effect_dynamics/2, starmac_motor_vertical_effect_dynamics1/2, starmac_motor_vertical_effect_dynamics3/2, starmac_motor_vertical_effect_dynamics2/2
  starmac_motor_vertical_effect_dynamics3/1 -> Mux/4
  starmac_motor_vertical_effect_dynamics2/1 -> Mux/3
  starmac_motor_vertical_effect_dynamics1/1 -> Mux/2
  starmac_motor_vertical_effect_dynamics/1 -> Mux/1
  Demux/4 -> starmac_motor_vertical_effect_dynamics3/1
  Demux/3 -> starmac_motor_vertical_effect_dynamics2/1
  Demux/2 -> starmac_motor_vertical_effect_dynamics1/1
  Demux/1 -> starmac_motor_vertical_effect_dynamics/1
  Mux/1 -> thrust_multiplier/1
  motor_thrusts/1 -> Demux/1

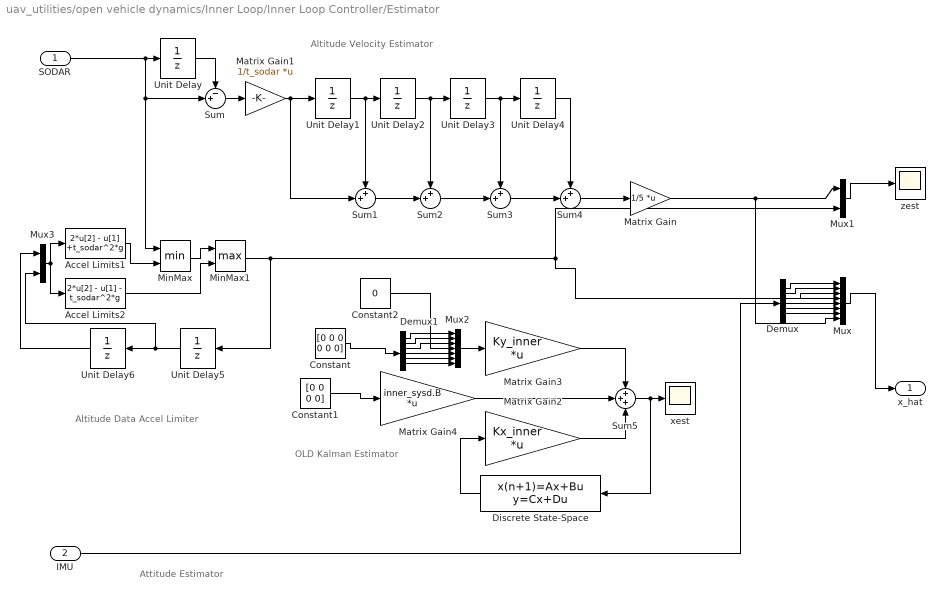
== system uav_utilities/open vehicle dynamics/Inner Loop/Inner Loop Controller/Estimator ==
  note: Altitude Velocity Estimator
  note: Attitude Estimator
  note: Altitude Data
      | Accel Limiter
  note: OLD
      | Kalman Estimator
  SODAR : Inport  PortDimensions=1  OutDataType=sfix(16)  OutScaling=2^0
  IMU : Inport  Port=2  OutDataType=sfix(16)  OutScaling=2^0
  Accel Limits1 : Fcn  Expr=2*u[2] - u[1] +t_sodar^2*g
  Accel Limits2 : Fcn  Expr=2*u[2] - u[1] - t_sodar^2*g
  Constant : Constant  Value=[0 0 0 0 0 0]  OutDataType=sfix(16)  OutScaling=2^0
  Constant1 : Constant  Value=[0 0 0 0]  OutDataType=sfix(16)  OutScaling=2^0
  Constant2 : Constant  Value=0  OutDataType=sfix(16)  OutScaling=2^0
  Demux : Demux  Outputs=6
  Demux1 : Demux  Outputs=6
  Discrete State-Space : DiscreteStateSpace  Orientation=left  A=zeros(8)  B=eye(8)  C=eye(8)  D=zeros(8)  X0=zeros(8,1)  SampleTime=t_imu
  Matrix Gain : Gain  Gain=1/5  Multiplication=Matrix(K*u)  ParameterDataType=sfix(16)  ParameterScaling=2^0  OutDataType=sfix(16)  OutScaling=2^0  SaturateOnIntegerOverflow=on  OutDataTypeStr=Inherit: Same as input  ParamDataTypeStr=Inherit: Same as input
  Matrix Gain1 : Gain  Gain=1/t_sodar  Multiplication=Matrix(K*u)  ParameterDataType=sfix(16)  ParameterScaling=2^0  OutDataType=sfix(16)  OutScaling=2^0  SaturateOnIntegerOverflow=on  OutDataTypeStr=Inherit: Same as input  ParamDataTypeStr=Inherit: Same as input
  Matrix Gain2 : Gain  Gain=Kx_inner  Multiplication=Matrix(K*u)  ParameterDataType=sfix(16)  ParameterScaling=2^0  OutDataType=sfix(16)  OutScaling=2^0  SaturateOnIntegerOverflow=on  OutDataTypeStr=Inherit: Same as input  ParamDataTypeStr=Inherit: Same as input
  Matrix Gain3 : Gain  Gain=Ky_inner  Multiplication=Matrix(K*u)  ParameterDataType=sfix(16)  ParameterScaling=2^0  OutDataType=sfix(16)  OutScaling=2^0  SaturateOnIntegerOverflow=on  OutDataTypeStr=Inherit: Same as input  ParamDataTypeStr=Inherit: Same as input
  Matrix Gain4 : Gain  Gain=inner_sysd.B  Multiplication=Matrix(K*u)  ParameterDataType=sfix(16)  ParameterScaling=2^0  OutDataType=sfix(16)  OutScaling=2^0  SaturateOnIntegerOverflow=on  OutDataTypeStr=Inherit: Same as input  ParamDataTypeStr=Inherit: Same as input
  MinMax : MinMax  Inputs=2  OutDataType=sfix(16)  OutScaling=2^0  SaturateOnIntegerOverflow=on  InputSameDT=on
  MinMax1 : MinMax  Function=max  Inputs=2  OutDataType=sfix(16)  OutScaling=2^0  SaturateOnIntegerOverflow=on  InputSameDT=on
  Mux : Mux  Inputs=8
  Mux1 : Mux  Inputs=2
  Mux2 : Mux  Inputs=7
  Mux3 : Mux  Inputs=2
  Sum : Sum  Inputs=-+|  OutDataType=sfix(16)  OutScaling=2^0  SaturateOnIntegerOverflow=on
  Sum{1..4} (4 alike) : Sum  Inputs=++|  OutDataType=sfix(16)  OutScaling=2^0  SaturateOnIntegerOverflow=on
  Sum5 : Sum  Inputs=+++  OutDataType=sfix(16)  OutScaling=2^0  SaturateOnIntegerOverflow=on
  Unit Delay{,1..4} (5 alike) : UnitDelay  SampleTime=t_sodar
  Unit Delay5 : UnitDelay  Orientation=left  SampleTime=t_sodar
  Unit Delay6 : UnitDelay  Orientation=left  SampleTime=t_sodar
  xest : Scope
      settings: SaveName=ScopeData8
  zest : Scope
      settings: YMin=-0.25  YMax=3.5  SaveName=ScopeData5
  x_hat : Outport  OutDataType=sfix(16)  OutScaling=2^0
  wires:
  Mux/1 -> x_hat/1
  IMU/1 -> Demux/1
  Demux/1 -> Mux/1
  Demux/2 -> Mux/2
  Demux/3 -> Mux/3
  Demux/4 -> Mux/5
  Demux/5 -> Mux/6
  Demux/6 -> Mux/7
  Unit Delay1/1 -> Sum1/1, Unit Delay2/1
  Unit Delay2/1 -> Unit Delay3/1, Sum2/1
  Unit Delay3/1 -> Unit Delay4/1, Sum3/1
  Unit Delay4/1 -> Sum4/1
  Sum1/1 -> Sum2/2
  Sum2/1 -> Sum3/2
  Sum3/1 -> Sum4/2
  Sum4/1 -> Matrix Gain/1
  Unit Delay/1 -> Sum/1
  SODAR/1 -> Unit Delay/1, Sum/2, MinMax/1
  Sum/1 -> Matrix Gain1/1
  Matrix Gain1/1 -> Unit Delay1/1, Sum1/2
  Matrix Gain/1 -> Mux/8, Mux1/1
  Mux1/1 -> zest/1
  MinMax1/1 -> Mux/4, Mux1/2, Unit Delay5/1
  Unit Delay5/1 -> Unit Delay6/1, Mux3/2
  Unit Delay6/1 -> Mux3/1
  Mux3/1 -> Accel Limits1/1, Accel Limits2/1
  Accel Limits1/1 -> MinMax/2
  Accel Limits2/1 -> MinMax1/2
  MinMax/1 -> MinMax1/1
  Mux2/1 -> Matrix Gain3/1
  Matrix Gain3/1 -> Sum5/1
  Sum5/1 -> xest/1, Discrete State-Space/1
  Constant/1 -> Demux1/1
  Demux1/1 -> Mux2/1
  Demux1/2 -> Mux2/2
  Demux1/3 -> Mux2/3
  Demux1/4 -> Mux2/5
  Demux1/5 -> Mux2/6
  Demux1/6 -> Mux2/7
  Constant1/1 -> Matrix Gain4/1
  Matrix Gain2/1 -> Sum5/3
  Matrix Gain4/1 -> Sum5/2
  Discrete State-Space/1 -> Matrix Gain2/1
  Constant2/1 -> Mux2/4

== system uav_utilities/open vehicle dynamics/Inner Loop/Inner Loop Controller/Sensor Noise Model   ==
  Mux3 : Mux  Inputs=6
  phi White Noise : simulink/Sources/Band-Limited White Noise  SystemSampleTime=-1  Cov=[pow_imu_pos_sim]  Ts=t_imu  seed=[60]
  phi_dot White Noise : simulink/Sources/Band-Limited White Noise  SystemSampleTime=-1  Cov=[pow_imu_rate_sim]  Ts=t_imu  seed=[40000]
  psi White Noise : simulink/Sources/Band-Limited White Noise  SystemSampleTime=-1  Cov=[pow_imu_pos_sim]  Ts=t_imu  seed=[80000]
  psi_dot White Noise : simulink/Sources/Band-Limited White Noise  SystemSampleTime=-1  Cov=[pow_imu_rate_sim]  Ts=t_imu  seed=[29999]
  theta White Noise : simulink/Sources/Band-Limited White Noise  SystemSampleTime=-1  Cov=[pow_imu_pos_sim]  Ts=t_imu  seed=[5000]
  theta_dot White Noise : simulink/Sources/Band-Limited White Noise  SystemSampleTime=-1  Cov=[pow_imu_rate_sim]  Ts=t_imu  seed=[3340]
  z White Noise : simulink/Sources/Band-Limited White Noise  SystemSampleTime=-1  Cov=[pow_sodar_sim]  Ts=t_sodar  seed=[39393]
  z Noise : Outport  OutDataType=sfix(16)  OutScaling=2^0
  Attitude Noise : Outport  Port=2  OutDataType=sfix(16)  OutScaling=2^0
  wires:
  Mux3/1 -> Attitude Noise/1
  psi White Noise/1 -> Mux3/3
  theta White Noise/1 -> Mux3/2
  phi White Noise/1 -> Mux3/1
  psi_dot White Noise/1 -> Mux3/6
  theta_dot White Noise/1 -> Mux3/5
  phi_dot White Noise/1 -> Mux3/4
  z White Noise/1 -> z Noise/1

== system uav_utilities/open vehicle dynamics/Inner Loop/Non-Linear Dynamics/Motor Model ==
  Thrust Command 1-4 : Inport  OutDataType=sfix(16)  OutScaling=2^0
  Euler (rad) : Inport  Port=2  OutDataType=sfix(16)  OutScaling=2^0
  Demux : Demux  Outputs=3
  Demux1 : Demux
  Motor {1..4} (4 alike) : TransferFcn  Denominator=[tau 1]
  Mux1 : Mux  Inputs=3
  PWM to Thrust : Gain  Gain=thrust_max  ParameterDataType=sfix(16)  ParameterScaling=2^0  OutDataType=sfix(16)  OutScaling=2^0  SaturateOnIntegerOverflow=on  OutDataTypeStr=Inherit: Same as input  ParamDataTypeStr=Inherit: Same as input
  Pitch Coupling : Product  OutDataType=sfix(16)  OutScaling=2^0  SaturateOnIntegerOverflow=on  OutDataTypeStr=Inherit: Same as first input
  RHCS : Gain  Gain=-1  ParameterDataType=sfix(16)  ParameterScaling=2^0  OutDataType=sfix(16)  OutScaling=2^0  SaturateOnIntegerOverflow=on  OutDataTypeStr=Inherit: Same as input  ParamDataTypeStr=Inherit: Same as input
  Roll Coupling : Product  OutDataType=sfix(16)  OutScaling=2^0  SaturateOnIntegerOverflow=on  OutDataTypeStr=Inherit: Same as first input
  Sum : Sum  Inputs=++++  OutDataType=sfix(16)  OutScaling=2^0  SaturateOnIntegerOverflow=on
  Terminator : Terminator
  Trigonometric Function : Trigonometry
  "Force_b " : Outport  OutDataType=sfix(16)  OutScaling=2^0
  wires:
  Demux1/1 -> Motor 1/1
  Demux1/4 -> Motor 4/1
  Demux1/2 -> Motor 2/1
  Sum/1 -> Pitch Coupling/1, Roll Coupling/1, Mux1/3
  Mux1/1 -> "Force_b "/1
  Euler (rad)/1 -> Trigonometric Function/1
  Pitch Coupling/1 -> RHCS/1
  Trigonometric Function/1 -> Demux/1
  Demux/1 -> Roll Coupling/2
  Demux/2 -> Pitch Coupling/2
  Demux/3 -> Terminator/1
  PWM to Thrust/1 -> Demux1/1
  Thrust Command 1-4/1 -> PWM to Thrust/1
  RHCS/1 -> Mux1/1
  Roll Coupling/1 -> Mux1/2
  Motor 1/1 -> Sum/1
  Motor 2/1 -> Sum/2
  Motor 4/1 -> Sum/4
  Demux1/3 -> Motor 3/1
  Motor 3/1 -> Sum/3

== system uav_utilities/open vehicle dynamics/Inner Loop/Non-Linear Dynamics/Rotational Torques ==
  Thrust Command 1-4 : Inport  OutDataType=sfix(16)  OutScaling=2^0
  Demux : Demux
  Matrix Gain : Gain  Gain=[[0,-L,0,L;L,0,-L,0]*thrust_max;[1,-1,1,-1]*torque_max]  Multiplication=Matrix(K*u)  ParameterDataType=sfix(16)  ParameterScaling=2^0  OutDataType=sfix(16)  OutScaling=2^0  SaturateOnIntegerOverflow=on  OutDataTypeStr=Inherit: Same as input  ParamDataTypeStr=Inherit: Same as input
  Motor {1..4} (4 alike) : TransferFcn  Denominator=[tau 1]
  Mux : Mux
  Moments : Outport  OutDataType=sfix(16)  OutScaling=2^0
  wires:
  Matrix Gain/1 -> Moments/1
  Thrust Command 1-4/1 -> Demux/1
  Demux/1 -> Motor 1/1
  Demux/2 -> Motor 2/1
  Demux/3 -> Motor 3/1
  Demux/4 -> Motor 4/1
  Motor 1/1 -> Mux/1
  Motor 2/1 -> Mux/2
  Motor 3/1 -> Mux/3
  Motor 4/1 -> Mux/4
  Mux/1 -> Matrix Gain/1

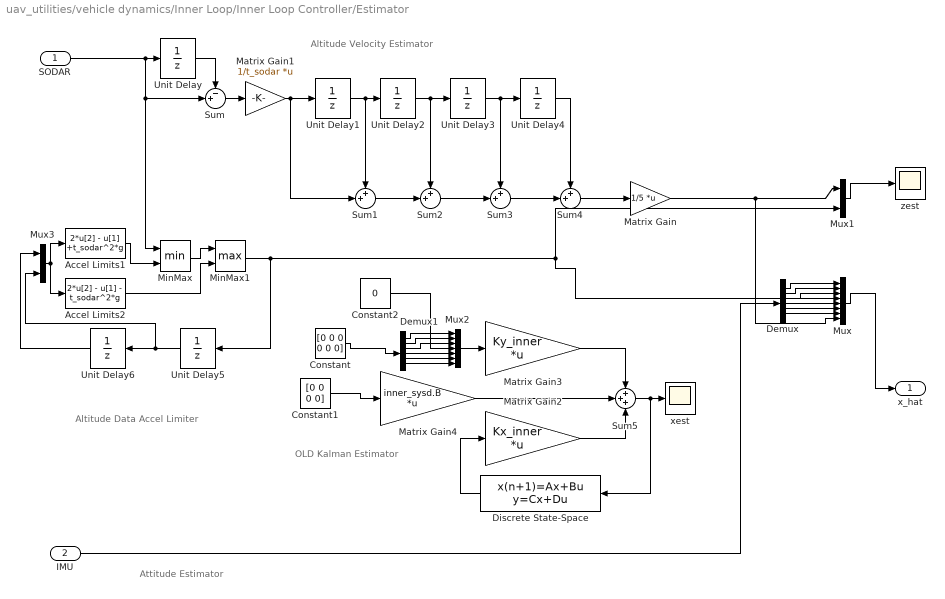
== system uav_utilities/vehicle dynamics/Inner Loop/Inner Loop Controller/Estimator ==
  note: OLD
      | Kalman Estimator
  note: Altitude Data
      | Accel Limiter
  note: Attitude Estimator
  note: Altitude Velocity Estimator
  SODAR : Inport  PortDimensions=1
  IMU : Inport  Port=2
  Accel Limits1 : Fcn  Expr=2*u[2] - u[1] +t_sodar^2*g
  Accel Limits2 : Fcn  Expr=2*u[2] - u[1] - t_sodar^2*g
  Constant : Constant  Value=[0 0 0 0 0 0]
  Constant1 : Constant  Value=[0 0 0 0]
  Constant2 : Constant  Value=0
  Demux : Demux  Outputs=6
  Demux1 : Demux  Outputs=6
  Discrete State-Space : DiscreteStateSpace  Orientation=left  A=zeros(8)  B=eye(8)  C=eye(8)  D=zeros(8)  X0=zeros(8,1)  SampleTime=t_imu
  Matrix Gain : Gain  Gain=1/5  Multiplication=Matrix(K*u)  SaturateOnIntegerOverflow=on  OutDataTypeStr=Inherit: Same as input  ParamDataTypeStr=Inherit: Same as input
  Matrix Gain1 : Gain  Gain=1/t_sodar  Multiplication=Matrix(K*u)  SaturateOnIntegerOverflow=on  OutDataTypeStr=Inherit: Same as input  ParamDataTypeStr=Inherit: Same as input
  Matrix Gain2 : Gain  Gain=Kx_inner  Multiplication=Matrix(K*u)  SaturateOnIntegerOverflow=on  OutDataTypeStr=Inherit: Same as input  ParamDataTypeStr=Inherit: Same as input
  Matrix Gain3 : Gain  Gain=Ky_inner  Multiplication=Matrix(K*u)  SaturateOnIntegerOverflow=on  OutDataTypeStr=Inherit: Same as input  ParamDataTypeStr=Inherit: Same as input
  Matrix Gain4 : Gain  Gain=inner_sysd.B  Multiplication=Matrix(K*u)  SaturateOnIntegerOverflow=on  OutDataTypeStr=Inherit: Same as input  ParamDataTypeStr=Inherit: Same as input
  MinMax : MinMax  Inputs=2  SaturateOnIntegerOverflow=on  InputSameDT=on
  MinMax1 : MinMax  Function=max  Inputs=2  SaturateOnIntegerOverflow=on  InputSameDT=on
  Mux : Mux  Inputs=8
  Mux1 : Mux  Inputs=2
  Mux2 : Mux  Inputs=7
  Mux3 : Mux  Inputs=2
  Sum : Sum  Inputs=-+|  SaturateOnIntegerOverflow=on
  Sum{1..4} (4 alike) : Sum  Inputs=++|  SaturateOnIntegerOverflow=on
  Sum5 : Sum  Inputs=+++  SaturateOnIntegerOverflow=on
  Unit Delay{,1..4} (5 alike) : UnitDelay  SampleTime=t_sodar
  Unit Delay5 : UnitDelay  Orientation=left  SampleTime=t_sodar
  Unit Delay6 : UnitDelay  Orientation=left  SampleTime=t_sodar
  xest : Scope
      settings: SaveName=ScopeData8
  zest : Scope
      settings: YMin=-0.25  YMax=3.5  SaveName=ScopeData5
  x_hat : Outport
  wires:
  Constant2/1 -> Mux2/4
  Discrete State-Space/1 -> Matrix Gain2/1
  Matrix Gain4/1 -> Sum5/2
  Matrix Gain2/1 -> Sum5/3
  Constant1/1 -> Matrix Gain4/1
  Demux1/6 -> Mux2/7
  Demux1/5 -> Mux2/6
  Demux1/4 -> Mux2/5
  Demux1/3 -> Mux2/3
  Demux1/2 -> Mux2/2
  Demux1/1 -> Mux2/1
  Constant/1 -> Demux1/1
  Sum5/1 -> Discrete State-Space/1, xest/1
  Matrix Gain3/1 -> Sum5/1
  Mux2/1 -> Matrix Gain3/1
  MinMax/1 -> MinMax1/1
  Accel Limits2/1 -> MinMax1/2
  Accel Limits1/1 -> MinMax/2
  Mux3/1 -> Accel Limits2/1, Accel Limits1/1
  Unit Delay6/1 -> Mux3/1
  Unit Delay5/1 -> Mux3/2, Unit Delay6/1
  MinMax1/1 -> Unit Delay5/1, Mux1/2, Mux/4
  Mux1/1 -> zest/1
  Matrix Gain/1 -> Mux1/1, Mux/8
  Matrix Gain1/1 -> Sum1/2, Unit Delay1/1
  Sum/1 -> Matrix Gain1/1
  SODAR/1 -> MinMax/1, Sum/2, Unit Delay/1
  Unit Delay/1 -> Sum/1
  Sum4/1 -> Matrix Gain/1
  Sum3/1 -> Sum4/2
  Sum2/1 -> Sum3/2
  Sum1/1 -> Sum2/2
  Unit Delay4/1 -> Sum4/1
  Unit Delay3/1 -> Sum3/1, Unit Delay4/1
  Unit Delay2/1 -> Sum2/1, Unit Delay3/1
  Unit Delay1/1 -> Unit Delay2/1, Sum1/1
  Demux/6 -> Mux/7
  Demux/5 -> Mux/6
  Demux/4 -> Mux/5
  Demux/3 -> Mux/3
  Demux/2 -> Mux/2
  Demux/1 -> Mux/1
  IMU/1 -> Demux/1
  Mux/1 -> x_hat/1

== system uav_utilities/vehicle dynamics/Inner Loop/Inner Loop Controller/Sensor Noise Model   ==
  Mux3 : Mux  Inputs=6
  phi White Noise : simulink/Sources/Band-Limited White Noise  SystemSampleTime=-1  Cov=[pow_imu_pos_sim]  Ts=t_imu  seed=[60]
  phi_dot White Noise : simulink/Sources/Band-Limited White Noise  SystemSampleTime=-1  Cov=[pow_imu_rate_sim]  Ts=t_imu  seed=[40000]
  psi White Noise : simulink/Sources/Band-Limited White Noise  SystemSampleTime=-1  Cov=[pow_imu_pos_sim]  Ts=t_imu  seed=[80000]
  psi_dot White Noise : simulink/Sources/Band-Limited White Noise  SystemSampleTime=-1  Cov=[pow_imu_rate_sim]  Ts=t_imu  seed=[29999]
  theta White Noise : simulink/Sources/Band-Limited White Noise  SystemSampleTime=-1  Cov=[pow_imu_pos_sim]  Ts=t_imu  seed=[5000]
  theta_dot White Noise : simulink/Sources/Band-Limited White Noise  SystemSampleTime=-1  Cov=[pow_imu_rate_sim]  Ts=t_imu  seed=[3340]
  z White Noise : simulink/Sources/Band-Limited White Noise  SystemSampleTime=-1  Cov=[pow_sodar_sim]  Ts=t_sodar  seed=[39393]
  z Noise : Outport
  Attitude Noise : Outport  Port=2
  wires:
  z White Noise/1 -> z Noise/1
  phi_dot White Noise/1 -> Mux3/4
  theta_dot White Noise/1 -> Mux3/5
  psi_dot White Noise/1 -> Mux3/6
  phi White Noise/1 -> Mux3/1
  theta White Noise/1 -> Mux3/2
  psi White Noise/1 -> Mux3/3
  Mux3/1 -> Attitude Noise/1

== system uav_utilities/vehicle dynamics/Inner Loop/Non-Linear Dynamics/Motor Model ==
  Thrust Command 1-4 : Inport
  Euler (rad) : Inport  Port=2
  Demux : Demux  Outputs=3
  Demux1 : Demux
  Motor {1..4} (4 alike) : TransferFcn  Denominator=[tau 1]
  Mux1 : Mux  Inputs=3
  PWM to Thrust : Gain  Gain=thrust_max  SaturateOnIntegerOverflow=on  OutDataTypeStr=Inherit: Same as input  ParamDataTypeStr=Inherit: Same as input
  Pitch Coupling : Product  SaturateOnIntegerOverflow=on  OutDataTypeStr=Inherit: Same as first input
  RHCS : Gain  Gain=-1  SaturateOnIntegerOverflow=on  OutDataTypeStr=Inherit: Same as input  ParamDataTypeStr=Inherit: Same as input
  Roll Coupling : Product  SaturateOnIntegerOverflow=on  OutDataTypeStr=Inherit: Same as first input
  Sum : Sum  Inputs=++++  SaturateOnIntegerOverflow=on
  Terminator : Terminator
  Trigonometric Function : Trigonometry
  "Force_b " : Outport
  wires:
  Motor 3/1 -> Sum/3
  Demux1/3 -> Motor 3/1
  Motor 4/1 -> Sum/4
  Motor 2/1 -> Sum/2
  Motor 1/1 -> Sum/1
  Roll Coupling/1 -> Mux1/2
  RHCS/1 -> Mux1/1
  Thrust Command 1-4/1 -> PWM to Thrust/1
  PWM to Thrust/1 -> Demux1/1
  Demux/3 -> Terminator/1
  Demux/2 -> Pitch Coupling/2
  Demux/1 -> Roll Coupling/2
  Trigonometric Function/1 -> Demux/1
  Pitch Coupling/1 -> RHCS/1
  Euler (rad)/1 -> Trigonometric Function/1
  Mux1/1 -> "Force_b "/1
  Sum/1 -> Mux1/3, Roll Coupling/1, Pitch Coupling/1
  Demux1/2 -> Motor 2/1
  Demux1/4 -> Motor 4/1
  Demux1/1 -> Motor 1/1

== system uav_utilities/vehicle dynamics/Inner Loop/Non-Linear Dynamics/Rotational Torques ==
  Thrust Command 1-4 : Inport
  Demux : Demux
  Matrix Gain : Gain  Gain=[[0,-L,0,L;L,0,-L,0]*thrust_max;[1,-1,1,-1]*torque_max]  Multiplication=Matrix(K*u)  SaturateOnIntegerOverflow=on  OutDataTypeStr=Inherit: Same as input  ParamDataTypeStr=Inherit: Same as input
  Motor {1..4} (4 alike) : TransferFcn  Denominator=[tau 1]
  Mux : Mux
  Moments : Outport
  wires:
  Mux/1 -> Matrix Gain/1
  Motor 4/1 -> Mux/4
  Motor 3/1 -> Mux/3
  Motor 2/1 -> Mux/2
  Motor 1/1 -> Mux/1
  Demux/4 -> Motor 4/1
  Demux/3 -> Motor 3/1
  Demux/2 -> Motor 2/1
  Demux/1 -> Motor 1/1
  Thrust Command 1-4/1 -> Demux/1
  Matrix Gain/1 -> Moments/1

== system uav_utilities/STARMAC/gum_stix/body_to_inertial/inertial_vel_and pos_est/DT_integrator ==
  Ab : Inport
  Sum : Sum  Inputs=++|  OutDataTypeMode=single  OutDataType=sfix(16)  OutScaling=2^0  OutDataTypeStr=single
  Sum1 : Sum  Inputs=|++  AccumDataTypeStr=single  OutDataType=sfix(16)  OutScaling=2^0
  negate : Gain  Gain=.5*Ts  ParameterDataType=sfix(16)  ParameterScaling=2^0  OutDataTypeMode=single  OutDataType=sfix(16)  OutScaling=2^0  OutDataTypeStr=single
  u_delay : UnitDelay  SampleTime=-1
  u_delay1 : UnitDelay  Orientation=left  SampleTime=-1
  Vb : Outport
  wires:
  u_delay1/1 -> Sum1/2
  Sum1/1 -> Vb/1, u_delay1/1
  negate/1 -> Sum1/1
  Sum/1 -> negate/1
  u_delay/1 -> Sum/1
  Ab/1 -> Sum/2, u_delay/1

== system uav_utilities/STARMAC/gum_stix/body_to_inertial/inertial_vel_and pos_est/DT_integrator1 ==
  Vb : Inport
  Sum : Sum  Inputs=++|  OutDataTypeMode=single  OutDataType=sfix(16)  OutScaling=2^0  OutDataTypeStr=single
  Sum1 : Sum  Inputs=|++  OutDataTypeMode=single  OutDataType=sfix(16)  OutScaling=2^0  OutDataTypeStr=single
  negate : Gain  Gain=.5*Ts  ParameterDataType=sfix(16)  ParameterScaling=2^0  OutDataTypeMode=single  OutDataType=sfix(16)  OutScaling=2^0  OutDataTypeStr=single
  u_delay : UnitDelay  SampleTime=-1
  u_delay1 : UnitDelay  Orientation=left  SampleTime=-1
  Xb : Outport  PortDimensions=[3]  DataType=single  OutDataTypeStr=single
  wires:
  Vb/1 -> u_delay/1, Sum/2
  u_delay/1 -> Sum/1
  Sum/1 -> negate/1
  negate/1 -> Sum1/1
  Sum1/1 -> u_delay1/1, Xb/1
  u_delay1/1 -> Sum1/2

== system uav_utilities/STARMAC/gum_stix/sensor_fusion/if_end/If Action Subsystem ==
  Xe_s : Inport  OutDataType=sfix(16)  OutScaling=2^0
  Xe_f : Inport  Port=2  OutDataType=sfix(16)  OutScaling=2^0
  Action Port : ActionPort  InitializeStates=reset
  Sum : Sum  Inputs=-+|  OutDataTypeMode=single  OutDataType=sfix(16)  OutScaling=2^0  OutDataTypeStr=single
  Xe_sh_1 : Outport  OutDataType=sfix(16)  OutScaling=2^0  OutputWhenDisabled=reset  InitialOutput=zeros(1,3,'single')
  dX_1 : Outport  Port=2  OutDataType=sfix(16)  OutScaling=2^0  OutputWhenDisabled=reset  InitialOutput=zeros(1,3,'single')
  wires:
  Sum/1 -> dX_1/1
  Xe_f/1 -> Sum/2
  Xe_s/1 -> Sum/1, Xe_sh_1/1
